simulink library "LibDBC_SCU_ch1"  (R2024b)
settings: Solver=VariableStepAuto  StartTime=0.0  StopTime=10.0  RelTol=1e-3
undefined symbols (not defined in the file): bit_packing, bit_unpacking, IO_Blk_Lib_TTC500, IO_CAN_ConfigMsg, IO_CAN_ReadMsg
libraries: simulink x59, IOBlock_Library_TTC580 x32
(part 20 of 21)

== system LibDBC_SCU_ch1/mBMS_Cell_Info_Slave2/IO_CAN_ReadMsg ==
  handle : Inport
  Enable : EnablePort
  IO_CAN_ReadMsg : IOBlock_Library_TTC580/CAN  Blocks TTC580 IOlib/ReadMsg_CAN/IO_CAN_ReadMsg  SampleTime=-1  ttlib=IO_Blk_Lib_TTC500  ttDescription=IO_CAN_ReadMsg  tt_iolib_version=0.19
      settings: SourceProductName=I/O Blocklibrary for TTC580
  ErrorCode : Outport  VectorParamsAs1DForOutWhenUnconnected=off
  buffer_data : Outport  Port=2  VectorParamsAs1DForOutWhenUnconnected=off
  buffer_length : Outport  Port=3  VectorParamsAs1DForOutWhenUnconnected=off
  buffer_id_format : Outport  Port=4  VectorParamsAs1DForOutWhenUnconnected=off
  buffer_id : Outport  Port=5  VectorParamsAs1DForOutWhenUnconnected=off
  wires:
  IO_CAN_ReadMsg/5 -> buffer_id/1
  IO_CAN_ReadMsg/4 -> buffer_id_format/1
  IO_CAN_ReadMsg/3 -> buffer_length/1
  IO_CAN_ReadMsg/2 -> buffer_data/1
  IO_CAN_ReadMsg/1 -> ErrorCode/1
  handle/1 -> IO_CAN_ReadMsg/1

== system LibDBC_SCU_ch1/mBMS_Cell_Info_Slave2/Trigger_Block ==
  Compare To Constant : simulink/Logic and Bit Operations/Compare To Constant  relop===  const=trigger_offset  OutDataTypeStr=boolean  ZeroCross=off
  Counter Limited : simulink/Sources/Counter Limited  uplimit=max(derate - 1,0)  tsamp=-1
  Trigger : Outport  VectorParamsAs1DForOutWhenUnconnected=off
  wires:
  Compare To Constant/1 -> Trigger/1
  Counter Limited/1 -> Compare To Constant/1

== system LibDBC_SCU_ch1/mBMS_Cell_Info_Slave2/bit_unpacking1 ==
  Data_in : Inport
  bit_unpacking_s : S-Function  FunctionName=bit_unpacking_s  Parameters=SampleTime,Endianness,Format,Inversion,Startbit,Width_bits,Factor,Offset  SFunctionDeploymentMode=off  EnableBusSupport=off
  Data_out : Outport  VectorParamsAs1DForOutWhenUnconnected=off
  wires:
  Data_in/1 -> bit_unpacking_s/1
  bit_unpacking_s/1 -> Data_out/1

== system LibDBC_SCU_ch1/mBMS_Cell_Info_Slave2/bit_unpacking2 ==
  Data_in : Inport
  bit_unpacking_s : S-Function  FunctionName=bit_unpacking_s  Parameters=SampleTime,Endianness,Format,Inversion,Startbit,Width_bits,Factor,Offset  SFunctionDeploymentMode=off  EnableBusSupport=off
  Data_out : Outport  VectorParamsAs1DForOutWhenUnconnected=off
  wires:
  Data_in/1 -> bit_unpacking_s/1
  bit_unpacking_s/1 -> Data_out/1

== system LibDBC_SCU_ch1/mBMS_Cell_Info_Slave2/bit_unpacking3 ==
  Data_in : Inport
  bit_unpacking_s : S-Function  FunctionName=bit_unpacking_s  Parameters=SampleTime,Endianness,Format,Inversion,Startbit,Width_bits,Factor,Offset  SFunctionDeploymentMode=off  EnableBusSupport=off
  Data_out : Outport  VectorParamsAs1DForOutWhenUnconnected=off
  wires:
  Data_in/1 -> bit_unpacking_s/1
  bit_unpacking_s/1 -> Data_out/1

== system LibDBC_SCU_ch1/mBMS_Cell_Info_Slave2/bit_unpacking4 ==
  Data_in : Inport
  bit_unpacking_s : S-Function  FunctionName=bit_unpacking_s  Parameters=SampleTime,Endianness,Format,Inversion,Startbit,Width_bits,Factor,Offset  SFunctionDeploymentMode=off  EnableBusSupport=off
  Data_out : Outport  VectorParamsAs1DForOutWhenUnconnected=off
  wires:
  Data_in/1 -> bit_unpacking_s/1
  bit_unpacking_s/1 -> Data_out/1

== system LibDBC_SCU_ch1/mBMS_Cell_Info_Slave2/bit_unpacking5 ==
  Data_in : Inport
  bit_unpacking_s : S-Function  FunctionName=bit_unpacking_s  Parameters=SampleTime,Endianness,Format,Inversion,Startbit,Width_bits,Factor,Offset  SFunctionDeploymentMode=off  EnableBusSupport=off
  Data_out : Outport  VectorParamsAs1DForOutWhenUnconnected=off
  wires:
  Data_in/1 -> bit_unpacking_s/1
  bit_unpacking_s/1 -> Data_out/1

== system LibDBC_SCU_ch1/mBMS_Cell_Info_Slave3/IO_CAN_ConfigMsg ==
  IO_CAN_ConfigMsg_s : S-Function  FunctionName=IO_CAN_ConfigMsg_s  Parameters=SampleTime,channel,mode,id_format,id,ac_mask  SFunctionDeploymentMode=off  EnableBusSupport=off
  ErrorCode : Outport  VectorParamsAs1DForOutWhenUnconnected=off
  handle : Outport  Port=2  VectorParamsAs1DForOutWhenUnconnected=off
  wires:
  IO_CAN_ConfigMsg_s/2 -> handle/1
  IO_CAN_ConfigMsg_s/1 -> ErrorCode/1

== system LibDBC_SCU_ch1/mBMS_Cell_Info_Slave3/IO_CAN_ReadMsg ==
  handle : Inport
  Enable : EnablePort
  IO_CAN_ReadMsg : IOBlock_Library_TTC580/CAN  Blocks TTC580 IOlib/ReadMsg_CAN/IO_CAN_ReadMsg  SampleTime=-1  ttlib=IO_Blk_Lib_TTC500  ttDescription=IO_CAN_ReadMsg  tt_iolib_version=0.19
      settings: SourceProductName=I/O Blocklibrary for TTC580
  ErrorCode : Outport  VectorParamsAs1DForOutWhenUnconnected=off
  buffer_data : Outport  Port=2  VectorParamsAs1DForOutWhenUnconnected=off
  buffer_length : Outport  Port=3  VectorParamsAs1DForOutWhenUnconnected=off
  buffer_id_format : Outport  Port=4  VectorParamsAs1DForOutWhenUnconnected=off
  buffer_id : Outport  Port=5  VectorParamsAs1DForOutWhenUnconnected=off
  wires:
  IO_CAN_ReadMsg/5 -> buffer_id/1
  IO_CAN_ReadMsg/4 -> buffer_id_format/1
  IO_CAN_ReadMsg/3 -> buffer_length/1
  IO_CAN_ReadMsg/2 -> buffer_data/1
  IO_CAN_ReadMsg/1 -> ErrorCode/1
  handle/1 -> IO_CAN_ReadMsg/1

== system LibDBC_SCU_ch1/mBMS_Cell_Info_Slave3/Trigger_Block ==
  Compare To Constant : simulink/Logic and Bit Operations/Compare To Constant  relop===  const=trigger_offset  OutDataTypeStr=boolean  ZeroCross=off
  Counter Limited : simulink/Sources/Counter Limited  uplimit=max(derate - 1,0)  tsamp=-1
  Trigger : Outport  VectorParamsAs1DForOutWhenUnconnected=off
  wires:
  Compare To Constant/1 -> Trigger/1
  Counter Limited/1 -> Compare To Constant/1

== system LibDBC_SCU_ch1/mBMS_Cell_Info_Slave3/bit_unpacking1 ==
  Data_in : Inport
  bit_unpacking_s : S-Function  FunctionName=bit_unpacking_s  Parameters=SampleTime,Endianness,Format,Inversion,Startbit,Width_bits,Factor,Offset  SFunctionDeploymentMode=off  EnableBusSupport=off
  Data_out : Outport  VectorParamsAs1DForOutWhenUnconnected=off
  wires:
  Data_in/1 -> bit_unpacking_s/1
  bit_unpacking_s/1 -> Data_out/1

== system LibDBC_SCU_ch1/mBMS_Cell_Info_Slave3/bit_unpacking2 ==
  Data_in : Inport
  bit_unpacking_s : S-Function  FunctionName=bit_unpacking_s  Parameters=SampleTime,Endianness,Format,Inversion,Startbit,Width_bits,Factor,Offset  SFunctionDeploymentMode=off  EnableBusSupport=off
  Data_out : Outport  VectorParamsAs1DForOutWhenUnconnected=off
  wires:
  Data_in/1 -> bit_unpacking_s/1
  bit_unpacking_s/1 -> Data_out/1

== system LibDBC_SCU_ch1/mBMS_Cell_Info_Slave3/bit_unpacking3 ==
  Data_in : Inport
  bit_unpacking_s : S-Function  FunctionName=bit_unpacking_s  Parameters=SampleTime,Endianness,Format,Inversion,Startbit,Width_bits,Factor,Offset  SFunctionDeploymentMode=off  EnableBusSupport=off
  Data_out : Outport  VectorParamsAs1DForOutWhenUnconnected=off
  wires:
  Data_in/1 -> bit_unpacking_s/1
  bit_unpacking_s/1 -> Data_out/1

== system LibDBC_SCU_ch1/mBMS_Cell_Info_Slave3/bit_unpacking4 ==
  Data_in : Inport
  bit_unpacking_s : S-Function  FunctionName=bit_unpacking_s  Parameters=SampleTime,Endianness,Format,Inversion,Startbit,Width_bits,Factor,Offset  SFunctionDeploymentMode=off  EnableBusSupport=off
  Data_out : Outport  VectorParamsAs1DForOutWhenUnconnected=off
  wires:
  Data_in/1 -> bit_unpacking_s/1
  bit_unpacking_s/1 -> Data_out/1

== system LibDBC_SCU_ch1/mBMS_Cell_Info_Slave3/bit_unpacking5 ==
  Data_in : Inport
  bit_unpacking_s : S-Function  FunctionName=bit_unpacking_s  Parameters=SampleTime,Endianness,Format,Inversion,Startbit,Width_bits,Factor,Offset  SFunctionDeploymentMode=off  EnableBusSupport=off
  Data_out : Outport  VectorParamsAs1DForOutWhenUnconnected=off
  wires:
  Data_in/1 -> bit_unpacking_s/1
  bit_unpacking_s/1 -> Data_out/1

== system LibDBC_SCU_ch1/mBMS_Cell_Info_Slave4/IO_CAN_ConfigMsg ==
  IO_CAN_ConfigMsg_s : S-Function  FunctionName=IO_CAN_ConfigMsg_s  Parameters=SampleTime,channel,mode,id_format,id,ac_mask  SFunctionDeploymentMode=off  EnableBusSupport=off
  ErrorCode : Outport  VectorParamsAs1DForOutWhenUnconnected=off
  handle : Outport  Port=2  VectorParamsAs1DForOutWhenUnconnected=off
  wires:
  IO_CAN_ConfigMsg_s/2 -> handle/1
  IO_CAN_ConfigMsg_s/1 -> ErrorCode/1

== system LibDBC_SCU_ch1/mBMS_Cell_Info_Slave4/IO_CAN_ReadMsg ==
  handle : Inport
  Enable : EnablePort
  IO_CAN_ReadMsg : IOBlock_Library_TTC580/CAN  Blocks TTC580 IOlib/ReadMsg_CAN/IO_CAN_ReadMsg  SampleTime=-1  ttlib=IO_Blk_Lib_TTC500  ttDescription=IO_CAN_ReadMsg  tt_iolib_version=0.19
      settings: SourceProductName=I/O Blocklibrary for TTC580
  ErrorCode : Outport  VectorParamsAs1DForOutWhenUnconnected=off
  buffer_data : Outport  Port=2  VectorParamsAs1DForOutWhenUnconnected=off
  buffer_length : Outport  Port=3  VectorParamsAs1DForOutWhenUnconnected=off
  buffer_id_format : Outport  Port=4  VectorParamsAs1DForOutWhenUnconnected=off
  buffer_id : Outport  Port=5  VectorParamsAs1DForOutWhenUnconnected=off
  wires:
  IO_CAN_ReadMsg/5 -> buffer_id/1
  IO_CAN_ReadMsg/4 -> buffer_id_format/1
  IO_CAN_ReadMsg/3 -> buffer_length/1
  IO_CAN_ReadMsg/2 -> buffer_data/1
  IO_CAN_ReadMsg/1 -> ErrorCode/1
  handle/1 -> IO_CAN_ReadMsg/1

== system LibDBC_SCU_ch1/mBMS_Cell_Info_Slave4/Trigger_Block ==
  Compare To Constant : simulink/Logic and Bit Operations/Compare To Constant  relop===  const=trigger_offset  OutDataTypeStr=boolean  ZeroCross=off
  Counter Limited : simulink/Sources/Counter Limited  uplimit=max(derate - 1,0)  tsamp=-1
  Trigger : Outport  VectorParamsAs1DForOutWhenUnconnected=off
  wires:
  Compare To Constant/1 -> Trigger/1
  Counter Limited/1 -> Compare To Constant/1

== system LibDBC_SCU_ch1/mBMS_Cell_Info_Slave4/bit_unpacking1 ==
  Data_in : Inport
  bit_unpacking_s : S-Function  FunctionName=bit_unpacking_s  Parameters=SampleTime,Endianness,Format,Inversion,Startbit,Width_bits,Factor,Offset  SFunctionDeploymentMode=off  EnableBusSupport=off
  Data_out : Outport  VectorParamsAs1DForOutWhenUnconnected=off
  wires:
  Data_in/1 -> bit_unpacking_s/1
  bit_unpacking_s/1 -> Data_out/1

== system LibDBC_SCU_ch1/mBMS_Cell_Info_Slave4/bit_unpacking2 ==
  Data_in : Inport
  bit_unpacking_s : S-Function  FunctionName=bit_unpacking_s  Parameters=SampleTime,Endianness,Format,Inversion,Startbit,Width_bits,Factor,Offset  SFunctionDeploymentMode=off  EnableBusSupport=off
  Data_out : Outport  VectorParamsAs1DForOutWhenUnconnected=off
  wires:
  Data_in/1 -> bit_unpacking_s/1
  bit_unpacking_s/1 -> Data_out/1

== system LibDBC_SCU_ch1/mBMS_Cell_Info_Slave4/bit_unpacking3 ==
  Data_in : Inport
  bit_unpacking_s : S-Function  FunctionName=bit_unpacking_s  Parameters=SampleTime,Endianness,Format,Inversion,Startbit,Width_bits,Factor,Offset  SFunctionDeploymentMode=off  EnableBusSupport=off
  Data_out : Outport  VectorParamsAs1DForOutWhenUnconnected=off
  wires:
  Data_in/1 -> bit_unpacking_s/1
  bit_unpacking_s/1 -> Data_out/1

== system LibDBC_SCU_ch1/mBMS_Cell_Info_Slave4/bit_unpacking4 ==
  Data_in : Inport
  bit_unpacking_s : S-Function  FunctionName=bit_unpacking_s  Parameters=SampleTime,Endianness,Format,Inversion,Startbit,Width_bits,Factor,Offset  SFunctionDeploymentMode=off  EnableBusSupport=off
  Data_out : Outport  VectorParamsAs1DForOutWhenUnconnected=off
  wires:
  Data_in/1 -> bit_unpacking_s/1
  bit_unpacking_s/1 -> Data_out/1

== system LibDBC_SCU_ch1/mBMS_Cell_Info_Slave4/bit_unpacking5 ==
  Data_in : Inport
  bit_unpacking_s : S-Function  FunctionName=bit_unpacking_s  Parameters=SampleTime,Endianness,Format,Inversion,Startbit,Width_bits,Factor,Offset  SFunctionDeploymentMode=off  EnableBusSupport=off
  Data_out : Outport  VectorParamsAs1DForOutWhenUnconnected=off
  wires:
  Data_in/1 -> bit_unpacking_s/1
  bit_unpacking_s/1 -> Data_out/1

== system LibDBC_SCU_ch1/mBMS_Cell_Info_Slave5/IO_CAN_ConfigMsg ==
  IO_CAN_ConfigMsg_s : S-Function  FunctionName=IO_CAN_ConfigMsg_s  Parameters=SampleTime,channel,mode,id_format,id,ac_mask  SFunctionDeploymentMode=off  EnableBusSupport=off
  ErrorCode : Outport  VectorParamsAs1DForOutWhenUnconnected=off
  handle : Outport  Port=2  VectorParamsAs1DForOutWhenUnconnected=off
  wires:
  IO_CAN_ConfigMsg_s/2 -> handle/1
  IO_CAN_ConfigMsg_s/1 -> ErrorCode/1

== system LibDBC_SCU_ch1/mBMS_Cell_Info_Slave5/IO_CAN_ReadMsg ==
  handle : Inport
  Enable : EnablePort
  IO_CAN_ReadMsg : IOBlock_Library_TTC580/CAN  Blocks TTC580 IOlib/ReadMsg_CAN/IO_CAN_ReadMsg  SampleTime=-1  ttlib=IO_Blk_Lib_TTC500  ttDescription=IO_CAN_ReadMsg  tt_iolib_version=0.19
      settings: SourceProductName=I/O Blocklibrary for TTC580
  ErrorCode : Outport  VectorParamsAs1DForOutWhenUnconnected=off
  buffer_data : Outport  Port=2  VectorParamsAs1DForOutWhenUnconnected=off
  buffer_length : Outport  Port=3  VectorParamsAs1DForOutWhenUnconnected=off
  buffer_id_format : Outport  Port=4  VectorParamsAs1DForOutWhenUnconnected=off
  buffer_id : Outport  Port=5  VectorParamsAs1DForOutWhenUnconnected=off
  wires:
  IO_CAN_ReadMsg/5 -> buffer_id/1
  IO_CAN_ReadMsg/4 -> buffer_id_format/1
  IO_CAN_ReadMsg/3 -> buffer_length/1
  IO_CAN_ReadMsg/2 -> buffer_data/1
  IO_CAN_ReadMsg/1 -> ErrorCode/1
  handle/1 -> IO_CAN_ReadMsg/1

== system LibDBC_SCU_ch1/mBMS_Cell_Info_Slave5/Trigger_Block ==
  Compare To Constant : simulink/Logic and Bit Operations/Compare To Constant  relop===  const=trigger_offset  OutDataTypeStr=boolean  ZeroCross=off
  Counter Limited : simulink/Sources/Counter Limited  uplimit=max(derate - 1,0)  tsamp=-1
  Trigger : Outport  VectorParamsAs1DForOutWhenUnconnected=off
  wires:
  Compare To Constant/1 -> Trigger/1
  Counter Limited/1 -> Compare To Constant/1

== system LibDBC_SCU_ch1/mBMS_Cell_Info_Slave5/bit_unpacking1 ==
  Data_in : Inport
  bit_unpacking_s : S-Function  FunctionName=bit_unpacking_s  Parameters=SampleTime,Endianness,Format,Inversion,Startbit,Width_bits,Factor,Offset  SFunctionDeploymentMode=off  EnableBusSupport=off
  Data_out : Outport  VectorParamsAs1DForOutWhenUnconnected=off
  wires:
  Data_in/1 -> bit_unpacking_s/1
  bit_unpacking_s/1 -> Data_out/1

== system LibDBC_SCU_ch1/mBMS_Cell_Info_Slave5/bit_unpacking2 ==
  Data_in : Inport
  bit_unpacking_s : S-Function  FunctionName=bit_unpacking_s  Parameters=SampleTime,Endianness,Format,Inversion,Startbit,Width_bits,Factor,Offset  SFunctionDeploymentMode=off  EnableBusSupport=off
  Data_out : Outport  VectorParamsAs1DForOutWhenUnconnected=off
  wires:
  Data_in/1 -> bit_unpacking_s/1
  bit_unpacking_s/1 -> Data_out/1

== system LibDBC_SCU_ch1/mBMS_Cell_Info_Slave5/bit_unpacking3 ==
  Data_in : Inport
  bit_unpacking_s : S-Function  FunctionName=bit_unpacking_s  Parameters=SampleTime,Endianness,Format,Inversion,Startbit,Width_bits,Factor,Offset  SFunctionDeploymentMode=off  EnableBusSupport=off
  Data_out : Outport  VectorParamsAs1DForOutWhenUnconnected=off
  wires:
  Data_in/1 -> bit_unpacking_s/1
  bit_unpacking_s/1 -> Data_out/1

== system LibDBC_SCU_ch1/mBMS_Cell_Info_Slave5/bit_unpacking4 ==
  Data_in : Inport
  bit_unpacking_s : S-Function  FunctionName=bit_unpacking_s  Parameters=SampleTime,Endianness,Format,Inversion,Startbit,Width_bits,Factor,Offset  SFunctionDeploymentMode=off  EnableBusSupport=off
  Data_out : Outport  VectorParamsAs1DForOutWhenUnconnected=off
  wires:
  Data_in/1 -> bit_unpacking_s/1
  bit_unpacking_s/1 -> Data_out/1

== system LibDBC_SCU_ch1/mBMS_Cell_Info_Slave5/bit_unpacking5 ==
  Data_in : Inport
  bit_unpacking_s : S-Function  FunctionName=bit_unpacking_s  Parameters=SampleTime,Endianness,Format,Inversion,Startbit,Width_bits,Factor,Offset  SFunctionDeploymentMode=off  EnableBusSupport=off
  Data_out : Outport  VectorParamsAs1DForOutWhenUnconnected=off
  wires:
  Data_in/1 -> bit_unpacking_s/1
  bit_unpacking_s/1 -> Data_out/1

== system LibDBC_SCU_ch1/mBMS_Cell_Info_Slave6/IO_CAN_ConfigMsg ==
  IO_CAN_ConfigMsg_s : S-Function  FunctionName=IO_CAN_ConfigMsg_s  Parameters=SampleTime,channel,mode,id_format,id,ac_mask  SFunctionDeploymentMode=off  EnableBusSupport=off
  ErrorCode : Outport  VectorParamsAs1DForOutWhenUnconnected=off
  handle : Outport  Port=2  VectorParamsAs1DForOutWhenUnconnected=off
  wires:
  IO_CAN_ConfigMsg_s/2 -> handle/1
  IO_CAN_ConfigMsg_s/1 -> ErrorCode/1

== system LibDBC_SCU_ch1/mBMS_Cell_Info_Slave6/IO_CAN_ReadMsg ==
  handle : Inport
  Enable : EnablePort
  IO_CAN_ReadMsg : IOBlock_Library_TTC580/CAN  Blocks TTC580 IOlib/ReadMsg_CAN/IO_CAN_ReadMsg  SampleTime=-1  ttlib=IO_Blk_Lib_TTC500  ttDescription=IO_CAN_ReadMsg  tt_iolib_version=0.19
      settings: SourceProductName=I/O Blocklibrary for TTC580
  ErrorCode : Outport  VectorParamsAs1DForOutWhenUnconnected=off
  buffer_data : Outport  Port=2  VectorParamsAs1DForOutWhenUnconnected=off
  buffer_length : Outport  Port=3  VectorParamsAs1DForOutWhenUnconnected=off
  buffer_id_format : Outport  Port=4  VectorParamsAs1DForOutWhenUnconnected=off
  buffer_id : Outport  Port=5  VectorParamsAs1DForOutWhenUnconnected=off
  wires:
  IO_CAN_ReadMsg/5 -> buffer_id/1
  IO_CAN_ReadMsg/4 -> buffer_id_format/1
  IO_CAN_ReadMsg/3 -> buffer_length/1
  IO_CAN_ReadMsg/2 -> buffer_data/1
  IO_CAN_ReadMsg/1 -> ErrorCode/1
  handle/1 -> IO_CAN_ReadMsg/1

== system LibDBC_SCU_ch1/mBMS_Cell_Info_Slave6/Trigger_Block ==
  Compare To Constant : simulink/Logic and Bit Operations/Compare To Constant  relop===  const=trigger_offset  OutDataTypeStr=boolean  ZeroCross=off
  Counter Limited : simulink/Sources/Counter Limited  uplimit=max(derate - 1,0)  tsamp=-1
  Trigger : Outport  VectorParamsAs1DForOutWhenUnconnected=off
  wires:
  Compare To Constant/1 -> Trigger/1
  Counter Limited/1 -> Compare To Constant/1

== system LibDBC_SCU_ch1/mBMS_Cell_Info_Slave6/bit_unpacking1 ==
  Data_in : Inport
  bit_unpacking_s : S-Function  FunctionName=bit_unpacking_s  Parameters=SampleTime,Endianness,Format,Inversion,Startbit,Width_bits,Factor,Offset  SFunctionDeploymentMode=off  EnableBusSupport=off
  Data_out : Outport  VectorParamsAs1DForOutWhenUnconnected=off
  wires:
  Data_in/1 -> bit_unpacking_s/1
  bit_unpacking_s/1 -> Data_out/1

== system LibDBC_SCU_ch1/mBMS_Cell_Info_Slave6/bit_unpacking2 ==
  Data_in : Inport
  bit_unpacking_s : S-Function  FunctionName=bit_unpacking_s  Parameters=SampleTime,Endianness,Format,Inversion,Startbit,Width_bits,Factor,Offset  SFunctionDeploymentMode=off  EnableBusSupport=off
  Data_out : Outport  VectorParamsAs1DForOutWhenUnconnected=off
  wires:
  Data_in/1 -> bit_unpacking_s/1
  bit_unpacking_s/1 -> Data_out/1

== system LibDBC_SCU_ch1/mBMS_Cell_Info_Slave6/bit_unpacking3 ==
  Data_in : Inport
  bit_unpacking_s : S-Function  FunctionName=bit_unpacking_s  Parameters=SampleTime,Endianness,Format,Inversion,Startbit,Width_bits,Factor,Offset  SFunctionDeploymentMode=off  EnableBusSupport=off
  Data_out : Outport  VectorParamsAs1DForOutWhenUnconnected=off
  wires:
  Data_in/1 -> bit_unpacking_s/1
  bit_unpacking_s/1 -> Data_out/1

== system LibDBC_SCU_ch1/mBMS_Cell_Info_Slave6/bit_unpacking4 ==
  Data_in : Inport
  bit_unpacking_s : S-Function  FunctionName=bit_unpacking_s  Parameters=SampleTime,Endianness,Format,Inversion,Startbit,Width_bits,Factor,Offset  SFunctionDeploymentMode=off  EnableBusSupport=off
  Data_out : Outport  VectorParamsAs1DForOutWhenUnconnected=off
  wires:
  Data_in/1 -> bit_unpacking_s/1
  bit_unpacking_s/1 -> Data_out/1

== system LibDBC_SCU_ch1/mBMS_Cell_Info_Slave6/bit_unpacking5 ==
  Data_in : Inport
  bit_unpacking_s : S-Function  FunctionName=bit_unpacking_s  Parameters=SampleTime,Endianness,Format,Inversion,Startbit,Width_bits,Factor,Offset  SFunctionDeploymentMode=off  EnableBusSupport=off
  Data_out : Outport  VectorParamsAs1DForOutWhenUnconnected=off
  wires:
  Data_in/1 -> bit_unpacking_s/1
  bit_unpacking_s/1 -> Data_out/1

== system LibDBC_SCU_ch1/mBMS_Cell_Info_Slave7/IO_CAN_ConfigMsg ==
  IO_CAN_ConfigMsg_s : S-Function  FunctionName=IO_CAN_ConfigMsg_s  Parameters=SampleTime,channel,mode,id_format,id,ac_mask  SFunctionDeploymentMode=off  EnableBusSupport=off
  ErrorCode : Outport  VectorParamsAs1DForOutWhenUnconnected=off
  handle : Outport  Port=2  VectorParamsAs1DForOutWhenUnconnected=off
  wires:
  IO_CAN_ConfigMsg_s/2 -> handle/1
  IO_CAN_ConfigMsg_s/1 -> ErrorCode/1

== system LibDBC_SCU_ch1/mBMS_Cell_Info_Slave7/IO_CAN_ReadMsg ==
  handle : Inport
  Enable : EnablePort
  IO_CAN_ReadMsg : IOBlock_Library_TTC580/CAN  Blocks TTC580 IOlib/ReadMsg_CAN/IO_CAN_ReadMsg  SampleTime=-1  ttlib=IO_Blk_Lib_TTC500  ttDescription=IO_CAN_ReadMsg  tt_iolib_version=0.19
      settings: SourceProductName=I/O Blocklibrary for TTC580
  ErrorCode : Outport  VectorParamsAs1DForOutWhenUnconnected=off
  buffer_data : Outport  Port=2  VectorParamsAs1DForOutWhenUnconnected=off
  buffer_length : Outport  Port=3  VectorParamsAs1DForOutWhenUnconnected=off
  buffer_id_format : Outport  Port=4  VectorParamsAs1DForOutWhenUnconnected=off
  buffer_id : Outport  Port=5  VectorParamsAs1DForOutWhenUnconnected=off
  wires:
  IO_CAN_ReadMsg/5 -> buffer_id/1
  IO_CAN_ReadMsg/4 -> buffer_id_format/1
  IO_CAN_ReadMsg/3 -> buffer_length/1
  IO_CAN_ReadMsg/2 -> buffer_data/1
  IO_CAN_ReadMsg/1 -> ErrorCode/1
  handle/1 -> IO_CAN_ReadMsg/1

== system LibDBC_SCU_ch1/mBMS_Cell_Info_Slave7/Trigger_Block ==
  Compare To Constant : simulink/Logic and Bit Operations/Compare To Constant  relop===  const=trigger_offset  OutDataTypeStr=boolean  ZeroCross=off
  Counter Limited : simulink/Sources/Counter Limited  uplimit=max(derate - 1,0)  tsamp=-1
  Trigger : Outport  VectorParamsAs1DForOutWhenUnconnected=off
  wires:
  Compare To Constant/1 -> Trigger/1
  Counter Limited/1 -> Compare To Constant/1

== system LibDBC_SCU_ch1/mBMS_Cell_Info_Slave7/bit_unpacking1 ==
  Data_in : Inport
  bit_unpacking_s : S-Function  FunctionName=bit_unpacking_s  Parameters=SampleTime,Endianness,Format,Inversion,Startbit,Width_bits,Factor,Offset  SFunctionDeploymentMode=off  EnableBusSupport=off
  Data_out : Outport  VectorParamsAs1DForOutWhenUnconnected=off
  wires:
  Data_in/1 -> bit_unpacking_s/1
  bit_unpacking_s/1 -> Data_out/1

== system LibDBC_SCU_ch1/mBMS_Cell_Info_Slave7/bit_unpacking2 ==
  Data_in : Inport
  bit_unpacking_s : S-Function  FunctionName=bit_unpacking_s  Parameters=SampleTime,Endianness,Format,Inversion,Startbit,Width_bits,Factor,Offset  SFunctionDeploymentMode=off  EnableBusSupport=off
  Data_out : Outport  VectorParamsAs1DForOutWhenUnconnected=off
  wires:
  Data_in/1 -> bit_unpacking_s/1
  bit_unpacking_s/1 -> Data_out/1

== system LibDBC_SCU_ch1/mBMS_Cell_Info_Slave7/bit_unpacking3 ==
  Data_in : Inport
  bit_unpacking_s : S-Function  FunctionName=bit_unpacking_s  Parameters=SampleTime,Endianness,Format,Inversion,Startbit,Width_bits,Factor,Offset  SFunctionDeploymentMode=off  EnableBusSupport=off
  Data_out : Outport  VectorParamsAs1DForOutWhenUnconnected=off
  wires:
  Data_in/1 -> bit_unpacking_s/1
  bit_unpacking_s/1 -> Data_out/1

== system LibDBC_SCU_ch1/mBMS_Cell_Info_Slave7/bit_unpacking4 ==
  Data_in : Inport
  bit_unpacking_s : S-Function  FunctionName=bit_unpacking_s  Parameters=SampleTime,Endianness,Format,Inversion,Startbit,Width_bits,Factor,Offset  SFunctionDeploymentMode=off  EnableBusSupport=off
  Data_out : Outport  VectorParamsAs1DForOutWhenUnconnected=off
  wires:
  Data_in/1 -> bit_unpacking_s/1
  bit_unpacking_s/1 -> Data_out/1

== system LibDBC_SCU_ch1/mBMS_Cell_Info_Slave7/bit_unpacking5 ==
  Data_in : Inport
  bit_unpacking_s : S-Function  FunctionName=bit_unpacking_s  Parameters=SampleTime,Endianness,Format,Inversion,Startbit,Width_bits,Factor,Offset  SFunctionDeploymentMode=off  EnableBusSupport=off
  Data_out : Outport  VectorParamsAs1DForOutWhenUnconnected=off
  wires:
  Data_in/1 -> bit_unpacking_s/1
  bit_unpacking_s/1 -> Data_out/1

== system LibDBC_SCU_ch1/mBMS_FuncSTAT/IO_CAN_ConfigMsg ==
  IO_CAN_ConfigMsg_s : S-Function  FunctionName=IO_CAN_ConfigMsg_s  Parameters=SampleTime,channel,mode,id_format,id,ac_mask  SFunctionDeploymentMode=off  EnableBusSupport=off
  ErrorCode : Outport  VectorParamsAs1DForOutWhenUnconnected=off
  handle : Outport  Port=2  VectorParamsAs1DForOutWhenUnconnected=off
  wires:
  IO_CAN_ConfigMsg_s/2 -> handle/1
  IO_CAN_ConfigMsg_s/1 -> ErrorCode/1

== system LibDBC_SCU_ch1/mBMS_FuncSTAT/IO_CAN_ReadMsg ==
  handle : Inport
  Enable : EnablePort
  IO_CAN_ReadMsg : IOBlock_Library_TTC580/CAN  Blocks TTC580 IOlib/ReadMsg_CAN/IO_CAN_ReadMsg  SampleTime=-1  ttlib=IO_Blk_Lib_TTC500  ttDescription=IO_CAN_ReadMsg  tt_iolib_version=0.19
      settings: SourceProductName=I/O Blocklibrary for TTC580
  ErrorCode : Outport  VectorParamsAs1DForOutWhenUnconnected=off
  buffer_data : Outport  Port=2  VectorParamsAs1DForOutWhenUnconnected=off
  buffer_length : Outport  Port=3  VectorParamsAs1DForOutWhenUnconnected=off
  buffer_id_format : Outport  Port=4  VectorParamsAs1DForOutWhenUnconnected=off
  buffer_id : Outport  Port=5  VectorParamsAs1DForOutWhenUnconnected=off
  wires:
  IO_CAN_ReadMsg/5 -> buffer_id/1
  IO_CAN_ReadMsg/4 -> buffer_id_format/1
  IO_CAN_ReadMsg/3 -> buffer_length/1
  IO_CAN_ReadMsg/2 -> buffer_data/1
  IO_CAN_ReadMsg/1 -> ErrorCode/1
  handle/1 -> IO_CAN_ReadMsg/1

== system LibDBC_SCU_ch1/mBMS_FuncSTAT/Trigger_Block ==
  Compare To Constant : simulink/Logic and Bit Operations/Compare To Constant  relop===  const=trigger_offset  OutDataTypeStr=boolean  ZeroCross=off
  Counter Limited : simulink/Sources/Counter Limited  uplimit=max(derate - 1,0)  tsamp=-1
  Trigger : Outport  VectorParamsAs1DForOutWhenUnconnected=off
  wires:
  Compare To Constant/1 -> Trigger/1
  Counter Limited/1 -> Compare To Constant/1

== system LibDBC_SCU_ch1/mBMS_FuncSTAT/bit_unpacking1 ==
  Data_in : Inport
  bit_unpacking_s : S-Function  FunctionName=bit_unpacking_s  Parameters=SampleTime,Endianness,Format,Inversion,Startbit,Width_bits,Factor,Offset  SFunctionDeploymentMode=off  EnableBusSupport=off
  Data_out : Outport  VectorParamsAs1DForOutWhenUnconnected=off
  wires:
  Data_in/1 -> bit_unpacking_s/1
  bit_unpacking_s/1 -> Data_out/1

== system LibDBC_SCU_ch1/mBMS_FuncSTAT/bit_unpacking10 ==
  Data_in : Inport
  bit_unpacking_s : S-Function  FunctionName=bit_unpacking_s  Parameters=SampleTime,Endianness,Format,Inversion,Startbit,Width_bits,Factor,Offset  SFunctionDeploymentMode=off  EnableBusSupport=off
  Data_out : Outport  VectorParamsAs1DForOutWhenUnconnected=off
  wires:
  Data_in/1 -> bit_unpacking_s/1
  bit_unpacking_s/1 -> Data_out/1

== system LibDBC_SCU_ch1/mBMS_FuncSTAT/bit_unpacking11 ==
  Data_in : Inport
  bit_unpacking_s : S-Function  FunctionName=bit_unpacking_s  Parameters=SampleTime,Endianness,Format,Inversion,Startbit,Width_bits,Factor,Offset  SFunctionDeploymentMode=off  EnableBusSupport=off
  Data_out : Outport  VectorParamsAs1DForOutWhenUnconnected=off
  wires:
  Data_in/1 -> bit_unpacking_s/1
  bit_unpacking_s/1 -> Data_out/1

== system LibDBC_SCU_ch1/mBMS_FuncSTAT/bit_unpacking12 ==
  Data_in : Inport
  bit_unpacking_s : S-Function  FunctionName=bit_unpacking_s  Parameters=SampleTime,Endianness,Format,Inversion,Startbit,Width_bits,Factor,Offset  SFunctionDeploymentMode=off  EnableBusSupport=off
  Data_out : Outport  VectorParamsAs1DForOutWhenUnconnected=off
  wires:
  Data_in/1 -> bit_unpacking_s/1
  bit_unpacking_s/1 -> Data_out/1

== system LibDBC_SCU_ch1/mBMS_FuncSTAT/bit_unpacking13 ==
  Data_in : Inport
  bit_unpacking_s : S-Function  FunctionName=bit_unpacking_s  Parameters=SampleTime,Endianness,Format,Inversion,Startbit,Width_bits,Factor,Offset  SFunctionDeploymentMode=off  EnableBusSupport=off
  Data_out : Outport  VectorParamsAs1DForOutWhenUnconnected=off
  wires:
  Data_in/1 -> bit_unpacking_s/1
  bit_unpacking_s/1 -> Data_out/1

== system LibDBC_SCU_ch1/mBMS_FuncSTAT/bit_unpacking14 ==
  Data_in : Inport
  bit_unpacking_s : S-Function  FunctionName=bit_unpacking_s  Parameters=SampleTime,Endianness,Format,Inversion,Startbit,Width_bits,Factor,Offset  SFunctionDeploymentMode=off  EnableBusSupport=off
  Data_out : Outport  VectorParamsAs1DForOutWhenUnconnected=off
  wires:
  Data_in/1 -> bit_unpacking_s/1
  bit_unpacking_s/1 -> Data_out/1

== system LibDBC_SCU_ch1/mBMS_FuncSTAT/bit_unpacking15 ==
  Data_in : Inport
  bit_unpacking_s : S-Function  FunctionName=bit_unpacking_s  Parameters=SampleTime,Endianness,Format,Inversion,Startbit,Width_bits,Factor,Offset  SFunctionDeploymentMode=off  EnableBusSupport=off
  Data_out : Outport  VectorParamsAs1DForOutWhenUnconnected=off
  wires:
  Data_in/1 -> bit_unpacking_s/1
  bit_unpacking_s/1 -> Data_out/1

== system LibDBC_SCU_ch1/mBMS_FuncSTAT/bit_unpacking16 ==
  Data_in : Inport
  bit_unpacking_s : S-Function  FunctionName=bit_unpacking_s  Parameters=SampleTime,Endianness,Format,Inversion,Startbit,Width_bits,Factor,Offset  SFunctionDeploymentMode=off  EnableBusSupport=off
  Data_out : Outport  VectorParamsAs1DForOutWhenUnconnected=off
  wires:
  Data_in/1 -> bit_unpacking_s/1
  bit_unpacking_s/1 -> Data_out/1

== system LibDBC_SCU_ch1/mBMS_FuncSTAT/bit_unpacking17 ==
  Data_in : Inport
  bit_unpacking_s : S-Function  FunctionName=bit_unpacking_s  Parameters=SampleTime,Endianness,Format,Inversion,Startbit,Width_bits,Factor,Offset  SFunctionDeploymentMode=off  EnableBusSupport=off
  Data_out : Outport  VectorParamsAs1DForOutWhenUnconnected=off
  wires:
  Data_in/1 -> bit_unpacking_s/1
  bit_unpacking_s/1 -> Data_out/1

== system LibDBC_SCU_ch1/mBMS_FuncSTAT/bit_unpacking18 ==
  Data_in : Inport
  bit_unpacking_s : S-Function  FunctionName=bit_unpacking_s  Parameters=SampleTime,Endianness,Format,Inversion,Startbit,Width_bits,Factor,Offset  SFunctionDeploymentMode=off  EnableBusSupport=off
  Data_out : Outport  VectorParamsAs1DForOutWhenUnconnected=off
  wires:
  Data_in/1 -> bit_unpacking_s/1
  bit_unpacking_s/1 -> Data_out/1

== system LibDBC_SCU_ch1/mBMS_FuncSTAT/bit_unpacking19 ==
  Data_in : Inport
  bit_unpacking_s : S-Function  FunctionName=bit_unpacking_s  Parameters=SampleTime,Endianness,Format,Inversion,Startbit,Width_bits,Factor,Offset  SFunctionDeploymentMode=off  EnableBusSupport=off
  Data_out : Outport  VectorParamsAs1DForOutWhenUnconnected=off
  wires:
  Data_in/1 -> bit_unpacking_s/1
  bit_unpacking_s/1 -> Data_out/1

== system LibDBC_SCU_ch1/mBMS_FuncSTAT/bit_unpacking2 ==
  Data_in : Inport
  bit_unpacking_s : S-Function  FunctionName=bit_unpacking_s  Parameters=SampleTime,Endianness,Format,Inversion,Startbit,Width_bits,Factor,Offset  SFunctionDeploymentMode=off  EnableBusSupport=off
  Data_out : Outport  VectorParamsAs1DForOutWhenUnconnected=off
  wires:
  Data_in/1 -> bit_unpacking_s/1
  bit_unpacking_s/1 -> Data_out/1

== system LibDBC_SCU_ch1/mBMS_FuncSTAT/bit_unpacking20 ==
  Data_in : Inport
  bit_unpacking_s : S-Function  FunctionName=bit_unpacking_s  Parameters=SampleTime,Endianness,Format,Inversion,Startbit,Width_bits,Factor,Offset  SFunctionDeploymentMode=off  EnableBusSupport=off
  Data_out : Outport  VectorParamsAs1DForOutWhenUnconnected=off
  wires:
  Data_in/1 -> bit_unpacking_s/1
  bit_unpacking_s/1 -> Data_out/1

== system LibDBC_SCU_ch1/mBMS_FuncSTAT/bit_unpacking21 ==
  Data_in : Inport
  bit_unpacking_s : S-Function  FunctionName=bit_unpacking_s  Parameters=SampleTime,Endianness,Format,Inversion,Startbit,Width_bits,Factor,Offset  SFunctionDeploymentMode=off  EnableBusSupport=off
  Data_out : Outport  VectorParamsAs1DForOutWhenUnconnected=off
  wires:
  Data_in/1 -> bit_unpacking_s/1
  bit_unpacking_s/1 -> Data_out/1

== system LibDBC_SCU_ch1/mBMS_FuncSTAT/bit_unpacking22 ==
  Data_in : Inport
  bit_unpacking_s : S-Function  FunctionName=bit_unpacking_s  Parameters=SampleTime,Endianness,Format,Inversion,Startbit,Width_bits,Factor,Offset  SFunctionDeploymentMode=off  EnableBusSupport=off
  Data_out : Outport  VectorParamsAs1DForOutWhenUnconnected=off
  wires:
  Data_in/1 -> bit_unpacking_s/1
  bit_unpacking_s/1 -> Data_out/1

== system LibDBC_SCU_ch1/mBMS_FuncSTAT/bit_unpacking23 ==
  Data_in : Inport
  bit_unpacking_s : S-Function  FunctionName=bit_unpacking_s  Parameters=SampleTime,Endianness,Format,Inversion,Startbit,Width_bits,Factor,Offset  SFunctionDeploymentMode=off  EnableBusSupport=off
  Data_out : Outport  VectorParamsAs1DForOutWhenUnconnected=off
  wires:
  Data_in/1 -> bit_unpacking_s/1
  bit_unpacking_s/1 -> Data_out/1

== system LibDBC_SCU_ch1/mBMS_FuncSTAT/bit_unpacking24 ==
  Data_in : Inport
  bit_unpacking_s : S-Function  FunctionName=bit_unpacking_s  Parameters=SampleTime,Endianness,Format,Inversion,Startbit,Width_bits,Factor,Offset  SFunctionDeploymentMode=off  EnableBusSupport=off
  Data_out : Outport  VectorParamsAs1DForOutWhenUnconnected=off
  wires:
  Data_in/1 -> bit_unpacking_s/1
  bit_unpacking_s/1 -> Data_out/1

== system LibDBC_SCU_ch1/mBMS_FuncSTAT/bit_unpacking25 ==
  Data_in : Inport
  bit_unpacking_s : S-Function  FunctionName=bit_unpacking_s  Parameters=SampleTime,Endianness,Format,Inversion,Startbit,Width_bits,Factor,Offset  SFunctionDeploymentMode=off  EnableBusSupport=off
  Data_out : Outport  VectorParamsAs1DForOutWhenUnconnected=off
  wires:
  Data_in/1 -> bit_unpacking_s/1
  bit_unpacking_s/1 -> Data_out/1

== system LibDBC_SCU_ch1/mBMS_FuncSTAT/bit_unpacking26 ==
  Data_in : Inport
  bit_unpacking_s : S-Function  FunctionName=bit_unpacking_s  Parameters=SampleTime,Endianness,Format,Inversion,Startbit,Width_bits,Factor,Offset  SFunctionDeploymentMode=off  EnableBusSupport=off
  Data_out : Outport  VectorParamsAs1DForOutWhenUnconnected=off
  wires:
  Data_in/1 -> bit_unpacking_s/1
  bit_unpacking_s/1 -> Data_out/1

== system LibDBC_SCU_ch1/mBMS_FuncSTAT/bit_unpacking27 ==
  Data_in : Inport
  bit_unpacking_s : S-Function  FunctionName=bit_unpacking_s  Parameters=SampleTime,Endianness,Format,Inversion,Startbit,Width_bits,Factor,Offset  SFunctionDeploymentMode=off  EnableBusSupport=off
  Data_out : Outport  VectorParamsAs1DForOutWhenUnconnected=off
  wires:
  Data_in/1 -> bit_unpacking_s/1
  bit_unpacking_s/1 -> Data_out/1

== system LibDBC_SCU_ch1/mBMS_FuncSTAT/bit_unpacking28 ==
  Data_in : Inport
  bit_unpacking_s : S-Function  FunctionName=bit_unpacking_s  Parameters=SampleTime,Endianness,Format,Inversion,Startbit,Width_bits,Factor,Offset  SFunctionDeploymentMode=off  EnableBusSupport=off
  Data_out : Outport  VectorParamsAs1DForOutWhenUnconnected=off
  wires:
  Data_in/1 -> bit_unpacking_s/1
  bit_unpacking_s/1 -> Data_out/1

== system LibDBC_SCU_ch1/mBMS_FuncSTAT/bit_unpacking29 ==
  Data_in : Inport
  bit_unpacking_s : S-Function  FunctionName=bit_unpacking_s  Parameters=SampleTime,Endianness,Format,Inversion,Startbit,Width_bits,Factor,Offset  SFunctionDeploymentMode=off  EnableBusSupport=off
  Data_out : Outport  VectorParamsAs1DForOutWhenUnconnected=off
  wires:
  Data_in/1 -> bit_unpacking_s/1
  bit_unpacking_s/1 -> Data_out/1

== system LibDBC_SCU_ch1/mBMS_FuncSTAT/bit_unpacking3 ==
  Data_in : Inport
  bit_unpacking_s : S-Function  FunctionName=bit_unpacking_s  Parameters=SampleTime,Endianness,Format,Inversion,Startbit,Width_bits,Factor,Offset  SFunctionDeploymentMode=off  EnableBusSupport=off
  Data_out : Outport  VectorParamsAs1DForOutWhenUnconnected=off
  wires:
  Data_in/1 -> bit_unpacking_s/1
  bit_unpacking_s/1 -> Data_out/1

== system LibDBC_SCU_ch1/mBMS_FuncSTAT/bit_unpacking30 ==
  Data_in : Inport
  bit_unpacking_s : S-Function  FunctionName=bit_unpacking_s  Parameters=SampleTime,Endianness,Format,Inversion,Startbit,Width_bits,Factor,Offset  SFunctionDeploymentMode=off  EnableBusSupport=off
  Data_out : Outport  VectorParamsAs1DForOutWhenUnconnected=off
  wires:
  Data_in/1 -> bit_unpacking_s/1
  bit_unpacking_s/1 -> Data_out/1

== system LibDBC_SCU_ch1/mBMS_FuncSTAT/bit_unpacking31 ==
  Data_in : Inport
  bit_unpacking_s : S-Function  FunctionName=bit_unpacking_s  Parameters=SampleTime,Endianness,Format,Inversion,Startbit,Width_bits,Factor,Offset  SFunctionDeploymentMode=off  EnableBusSupport=off
  Data_out : Outport  VectorParamsAs1DForOutWhenUnconnected=off
  wires:
  Data_in/1 -> bit_unpacking_s/1
  bit_unpacking_s/1 -> Data_out/1

== system LibDBC_SCU_ch1/mBMS_FuncSTAT/bit_unpacking32 ==
  Data_in : Inport
  bit_unpacking_s : S-Function  FunctionName=bit_unpacking_s  Parameters=SampleTime,Endianness,Format,Inversion,Startbit,Width_bits,Factor,Offset  SFunctionDeploymentMode=off  EnableBusSupport=off
  Data_out : Outport  VectorParamsAs1DForOutWhenUnconnected=off
  wires:
  Data_in/1 -> bit_unpacking_s/1
  bit_unpacking_s/1 -> Data_out/1

== system LibDBC_SCU_ch1/mBMS_FuncSTAT/bit_unpacking33 ==
  Data_in : Inport
  bit_unpacking_s : S-Function  FunctionName=bit_unpacking_s  Parameters=SampleTime,Endianness,Format,Inversion,Startbit,Width_bits,Factor,Offset  SFunctionDeploymentMode=off  EnableBusSupport=off
  Data_out : Outport  VectorParamsAs1DForOutWhenUnconnected=off
  wires:
  Data_in/1 -> bit_unpacking_s/1
  bit_unpacking_s/1 -> Data_out/1

== system LibDBC_SCU_ch1/mBMS_FuncSTAT/bit_unpacking34 ==
  Data_in : Inport
  bit_unpacking_s : S-Function  FunctionName=bit_unpacking_s  Parameters=SampleTime,Endianness,Format,Inversion,Startbit,Width_bits,Factor,Offset  SFunctionDeploymentMode=off  EnableBusSupport=off
  Data_out : Outport  VectorParamsAs1DForOutWhenUnconnected=off
  wires:
  Data_in/1 -> bit_unpacking_s/1
  bit_unpacking_s/1 -> Data_out/1

== system LibDBC_SCU_ch1/mBMS_FuncSTAT/bit_unpacking35 ==
  Data_in : Inport
  bit_unpacking_s : S-Function  FunctionName=bit_unpacking_s  Parameters=SampleTime,Endianness,Format,Inversion,Startbit,Width_bits,Factor,Offset  SFunctionDeploymentMode=off  EnableBusSupport=off
  Data_out : Outport  VectorParamsAs1DForOutWhenUnconnected=off
  wires:
  Data_in/1 -> bit_unpacking_s/1
  bit_unpacking_s/1 -> Data_out/1

== system LibDBC_SCU_ch1/mBMS_FuncSTAT/bit_unpacking36 ==
  Data_in : Inport
  bit_unpacking_s : S-Function  FunctionName=bit_unpacking_s  Parameters=SampleTime,Endianness,Format,Inversion,Startbit,Width_bits,Factor,Offset  SFunctionDeploymentMode=off  EnableBusSupport=off
  Data_out : Outport  VectorParamsAs1DForOutWhenUnconnected=off
  wires:
  Data_in/1 -> bit_unpacking_s/1
  bit_unpacking_s/1 -> Data_out/1

== system LibDBC_SCU_ch1/mBMS_FuncSTAT/bit_unpacking37 ==
  Data_in : Inport
  bit_unpacking_s : S-Function  FunctionName=bit_unpacking_s  Parameters=SampleTime,Endianness,Format,Inversion,Startbit,Width_bits,Factor,Offset  SFunctionDeploymentMode=off  EnableBusSupport=off
  Data_out : Outport  VectorParamsAs1DForOutWhenUnconnected=off
  wires:
  Data_in/1 -> bit_unpacking_s/1
  bit_unpacking_s/1 -> Data_out/1

== system LibDBC_SCU_ch1/mBMS_FuncSTAT/bit_unpacking38 ==
  Data_in : Inport
  bit_unpacking_s : S-Function  FunctionName=bit_unpacking_s  Parameters=SampleTime,Endianness,Format,Inversion,Startbit,Width_bits,Factor,Offset  SFunctionDeploymentMode=off  EnableBusSupport=off
  Data_out : Outport  VectorParamsAs1DForOutWhenUnconnected=off
  wires:
  Data_in/1 -> bit_unpacking_s/1
  bit_unpacking_s/1 -> Data_out/1

== system LibDBC_SCU_ch1/mBMS_FuncSTAT/bit_unpacking39 ==
  Data_in : Inport
  bit_unpacking_s : S-Function  FunctionName=bit_unpacking_s  Parameters=SampleTime,Endianness,Format,Inversion,Startbit,Width_bits,Factor,Offset  SFunctionDeploymentMode=off  EnableBusSupport=off
  Data_out : Outport  VectorParamsAs1DForOutWhenUnconnected=off
  wires:
  Data_in/1 -> bit_unpacking_s/1
  bit_unpacking_s/1 -> Data_out/1

== system LibDBC_SCU_ch1/mBMS_FuncSTAT/bit_unpacking4 ==
  Data_in : Inport
  bit_unpacking_s : S-Function  FunctionName=bit_unpacking_s  Parameters=SampleTime,Endianness,Format,Inversion,Startbit,Width_bits,Factor,Offset  SFunctionDeploymentMode=off  EnableBusSupport=off
  Data_out : Outport  VectorParamsAs1DForOutWhenUnconnected=off
  wires:
  Data_in/1 -> bit_unpacking_s/1
  bit_unpacking_s/1 -> Data_out/1

== system LibDBC_SCU_ch1/mBMS_FuncSTAT/bit_unpacking40 ==
  Data_in : Inport
  bit_unpacking_s : S-Function  FunctionName=bit_unpacking_s  Parameters=SampleTime,Endianness,Format,Inversion,Startbit,Width_bits,Factor,Offset  SFunctionDeploymentMode=off  EnableBusSupport=off
  Data_out : Outport  VectorParamsAs1DForOutWhenUnconnected=off
  wires:
  Data_in/1 -> bit_unpacking_s/1
  bit_unpacking_s/1 -> Data_out/1

== system LibDBC_SCU_ch1/mBMS_FuncSTAT/bit_unpacking41 ==
  Data_in : Inport
  bit_unpacking_s : S-Function  FunctionName=bit_unpacking_s  Parameters=SampleTime,Endianness,Format,Inversion,Startbit,Width_bits,Factor,Offset  SFunctionDeploymentMode=off  EnableBusSupport=off
  Data_out : Outport  VectorParamsAs1DForOutWhenUnconnected=off
  wires:
  Data_in/1 -> bit_unpacking_s/1
  bit_unpacking_s/1 -> Data_out/1

== system LibDBC_SCU_ch1/mBMS_FuncSTAT/bit_unpacking42 ==
  Data_in : Inport
  bit_unpacking_s : S-Function  FunctionName=bit_unpacking_s  Parameters=SampleTime,Endianness,Format,Inversion,Startbit,Width_bits,Factor,Offset  SFunctionDeploymentMode=off  EnableBusSupport=off
  Data_out : Outport  VectorParamsAs1DForOutWhenUnconnected=off
  wires:
  Data_in/1 -> bit_unpacking_s/1
  bit_unpacking_s/1 -> Data_out/1

== system LibDBC_SCU_ch1/mBMS_FuncSTAT/bit_unpacking43 ==
  Data_in : Inport
  bit_unpacking_s : S-Function  FunctionName=bit_unpacking_s  Parameters=SampleTime,Endianness,Format,Inversion,Startbit,Width_bits,Factor,Offset  SFunctionDeploymentMode=off  EnableBusSupport=off
  Data_out : Outport  VectorParamsAs1DForOutWhenUnconnected=off
  wires:
  Data_in/1 -> bit_unpacking_s/1
  bit_unpacking_s/1 -> Data_out/1

== system LibDBC_SCU_ch1/mBMS_FuncSTAT/bit_unpacking44 ==
  Data_in : Inport
  bit_unpacking_s : S-Function  FunctionName=bit_unpacking_s  Parameters=SampleTime,Endianness,Format,Inversion,Startbit,Width_bits,Factor,Offset  SFunctionDeploymentMode=off  EnableBusSupport=off
  Data_out : Outport  VectorParamsAs1DForOutWhenUnconnected=off
  wires:
  Data_in/1 -> bit_unpacking_s/1
  bit_unpacking_s/1 -> Data_out/1

== system LibDBC_SCU_ch1/mBMS_FuncSTAT/bit_unpacking5 ==
  Data_in : Inport
  bit_unpacking_s : S-Function  FunctionName=bit_unpacking_s  Parameters=SampleTime,Endianness,Format,Inversion,Startbit,Width_bits,Factor,Offset  SFunctionDeploymentMode=off  EnableBusSupport=off
  Data_out : Outport  VectorParamsAs1DForOutWhenUnconnected=off
  wires:
  Data_in/1 -> bit_unpacking_s/1
  bit_unpacking_s/1 -> Data_out/1

== system LibDBC_SCU_ch1/mBMS_FuncSTAT/bit_unpacking6 ==
  Data_in : Inport
  bit_unpacking_s : S-Function  FunctionName=bit_unpacking_s  Parameters=SampleTime,Endianness,Format,Inversion,Startbit,Width_bits,Factor,Offset  SFunctionDeploymentMode=off  EnableBusSupport=off
  Data_out : Outport  VectorParamsAs1DForOutWhenUnconnected=off
  wires:
  Data_in/1 -> bit_unpacking_s/1
  bit_unpacking_s/1 -> Data_out/1

== system LibDBC_SCU_ch1/mBMS_FuncSTAT/bit_unpacking7 ==
  Data_in : Inport
  bit_unpacking_s : S-Function  FunctionName=bit_unpacking_s  Parameters=SampleTime,Endianness,Format,Inversion,Startbit,Width_bits,Factor,Offset  SFunctionDeploymentMode=off  EnableBusSupport=off
  Data_out : Outport  VectorParamsAs1DForOutWhenUnconnected=off
  wires:
  Data_in/1 -> bit_unpacking_s/1
  bit_unpacking_s/1 -> Data_out/1

== system LibDBC_SCU_ch1/mBMS_FuncSTAT/bit_unpacking8 ==
  Data_in : Inport
  bit_unpacking_s : S-Function  FunctionName=bit_unpacking_s  Parameters=SampleTime,Endianness,Format,Inversion,Startbit,Width_bits,Factor,Offset  SFunctionDeploymentMode=off  EnableBusSupport=off
  Data_out : Outport  VectorParamsAs1DForOutWhenUnconnected=off
  wires:
  Data_in/1 -> bit_unpacking_s/1
  bit_unpacking_s/1 -> Data_out/1

== system LibDBC_SCU_ch1/mBMS_FuncSTAT/bit_unpacking9 ==
  Data_in : Inport
  bit_unpacking_s : S-Function  FunctionName=bit_unpacking_s  Parameters=SampleTime,Endianness,Format,Inversion,Startbit,Width_bits,Factor,Offset  SFunctionDeploymentMode=off  EnableBusSupport=off
  Data_out : Outport  VectorParamsAs1DForOutWhenUnconnected=off
  wires:
  Data_in/1 -> bit_unpacking_s/1
  bit_unpacking_s/1 -> Data_out/1

== system LibDBC_SCU_ch1/mBMS_PP/IO_CAN_ConfigMsg ==
  IO_CAN_ConfigMsg_s : S-Function  FunctionName=IO_CAN_ConfigMsg_s  Parameters=SampleTime,channel,mode,id_format,id,ac_mask  SFunctionDeploymentMode=off  EnableBusSupport=off
  ErrorCode : Outport  VectorParamsAs1DForOutWhenUnconnected=off
  handle : Outport  Port=2  VectorParamsAs1DForOutWhenUnconnected=off
  wires:
  IO_CAN_ConfigMsg_s/2 -> handle/1
  IO_CAN_ConfigMsg_s/1 -> ErrorCode/1

== system LibDBC_SCU_ch1/mBMS_PP/IO_CAN_ReadMsg ==
  handle : Inport
  Enable : EnablePort
  IO_CAN_ReadMsg : IOBlock_Library_TTC580/CAN  Blocks TTC580 IOlib/ReadMsg_CAN/IO_CAN_ReadMsg  SampleTime=-1  ttlib=IO_Blk_Lib_TTC500  ttDescription=IO_CAN_ReadMsg  tt_iolib_version=0.19
      settings: SourceProductName=I/O Blocklibrary for TTC580
  ErrorCode : Outport  VectorParamsAs1DForOutWhenUnconnected=off
  buffer_data : Outport  Port=2  VectorParamsAs1DForOutWhenUnconnected=off
  buffer_length : Outport  Port=3  VectorParamsAs1DForOutWhenUnconnected=off
  buffer_id_format : Outport  Port=4  VectorParamsAs1DForOutWhenUnconnected=off
  buffer_id : Outport  Port=5  VectorParamsAs1DForOutWhenUnconnected=off
  wires:
  IO_CAN_ReadMsg/5 -> buffer_id/1
  IO_CAN_ReadMsg/4 -> buffer_id_format/1
  IO_CAN_ReadMsg/3 -> buffer_length/1
  IO_CAN_ReadMsg/2 -> buffer_data/1
  IO_CAN_ReadMsg/1 -> ErrorCode/1
  handle/1 -> IO_CAN_ReadMsg/1

== system LibDBC_SCU_ch1/mBMS_PP/Trigger_Block ==
  Compare To Constant : simulink/Logic and Bit Operations/Compare To Constant  relop===  const=trigger_offset  OutDataTypeStr=boolean  ZeroCross=off
  Counter Limited : simulink/Sources/Counter Limited  uplimit=max(derate - 1,0)  tsamp=-1
  Trigger : Outport  VectorParamsAs1DForOutWhenUnconnected=off
  wires:
  Compare To Constant/1 -> Trigger/1
  Counter Limited/1 -> Compare To Constant/1

== system LibDBC_SCU_ch1/mBMS_PP/bit_unpacking1 ==
  Data_in : Inport
  bit_unpacking_s : S-Function  FunctionName=bit_unpacking_s  Parameters=SampleTime,Endianness,Format,Inversion,Startbit,Width_bits,Factor,Offset  SFunctionDeploymentMode=off  EnableBusSupport=off
  Data_out : Outport  VectorParamsAs1DForOutWhenUnconnected=off
  wires:
  Data_in/1 -> bit_unpacking_s/1
  bit_unpacking_s/1 -> Data_out/1

== system LibDBC_SCU_ch1/mBMS_PP/bit_unpacking2 ==
  Data_in : Inport
  bit_unpacking_s : S-Function  FunctionName=bit_unpacking_s  Parameters=SampleTime,Endianness,Format,Inversion,Startbit,Width_bits,Factor,Offset  SFunctionDeploymentMode=off  EnableBusSupport=off
  Data_out : Outport  VectorParamsAs1DForOutWhenUnconnected=off
  wires:
  Data_in/1 -> bit_unpacking_s/1
  bit_unpacking_s/1 -> Data_out/1

== system LibDBC_SCU_ch1/mBMS_PP/bit_unpacking3 ==
  Data_in : Inport
  bit_unpacking_s : S-Function  FunctionName=bit_unpacking_s  Parameters=SampleTime,Endianness,Format,Inversion,Startbit,Width_bits,Factor,Offset  SFunctionDeploymentMode=off  EnableBusSupport=off
  Data_out : Outport  VectorParamsAs1DForOutWhenUnconnected=off
  wires:
  Data_in/1 -> bit_unpacking_s/1
  bit_unpacking_s/1 -> Data_out/1

== system LibDBC_SCU_ch1/mBMS_PP/bit_unpacking4 ==
  Data_in : Inport
  bit_unpacking_s : S-Function  FunctionName=bit_unpacking_s  Parameters=SampleTime,Endianness,Format,Inversion,Startbit,Width_bits,Factor,Offset  SFunctionDeploymentMode=off  EnableBusSupport=off
  Data_out : Outport  VectorParamsAs1DForOutWhenUnconnected=off
  wires:
  Data_in/1 -> bit_unpacking_s/1
  bit_unpacking_s/1 -> Data_out/1

== system LibDBC_SCU_ch1/mBMS_RI_OCV_Approx/IO_CAN_ConfigMsg ==
  IO_CAN_ConfigMsg_s : S-Function  FunctionName=IO_CAN_ConfigMsg_s  Parameters=SampleTime,channel,mode,id_format,id,ac_mask  SFunctionDeploymentMode=off  EnableBusSupport=off
  ErrorCode : Outport  VectorParamsAs1DForOutWhenUnconnected=off
  handle : Outport  Port=2  VectorParamsAs1DForOutWhenUnconnected=off
  wires:
  IO_CAN_ConfigMsg_s/2 -> handle/1
  IO_CAN_ConfigMsg_s/1 -> ErrorCode/1

== system LibDBC_SCU_ch1/mBMS_RI_OCV_Approx/IO_CAN_ReadMsg ==
  handle : Inport
  Enable : EnablePort
  IO_CAN_ReadMsg : IOBlock_Library_TTC580/CAN  Blocks TTC580 IOlib/ReadMsg_CAN/IO_CAN_ReadMsg  SampleTime=-1  ttlib=IO_Blk_Lib_TTC500  ttDescription=IO_CAN_ReadMsg  tt_iolib_version=0.19
      settings: SourceProductName=I/O Blocklibrary for TTC580
  ErrorCode : Outport  VectorParamsAs1DForOutWhenUnconnected=off
  buffer_data : Outport  Port=2  VectorParamsAs1DForOutWhenUnconnected=off
  buffer_length : Outport  Port=3  VectorParamsAs1DForOutWhenUnconnected=off
  buffer_id_format : Outport  Port=4  VectorParamsAs1DForOutWhenUnconnected=off
  buffer_id : Outport  Port=5  VectorParamsAs1DForOutWhenUnconnected=off
  wires:
  IO_CAN_ReadMsg/5 -> buffer_id/1
  IO_CAN_ReadMsg/4 -> buffer_id_format/1
  IO_CAN_ReadMsg/3 -> buffer_length/1
  IO_CAN_ReadMsg/2 -> buffer_data/1
  IO_CAN_ReadMsg/1 -> ErrorCode/1
  handle/1 -> IO_CAN_ReadMsg/1

== system LibDBC_SCU_ch1/mBMS_RI_OCV_Approx/Trigger_Block ==
  Compare To Constant : simulink/Logic and Bit Operations/Compare To Constant  relop===  const=trigger_offset  OutDataTypeStr=boolean  ZeroCross=off
  Counter Limited : simulink/Sources/Counter Limited  uplimit=max(derate - 1,0)  tsamp=-1
  Trigger : Outport  VectorParamsAs1DForOutWhenUnconnected=off
  wires:
  Compare To Constant/1 -> Trigger/1
  Counter Limited/1 -> Compare To Constant/1

== system LibDBC_SCU_ch1/mBMS_RI_OCV_Approx/bit_unpacking1 ==
  Data_in : Inport
  bit_unpacking_s : S-Function  FunctionName=bit_unpacking_s  Parameters=SampleTime,Endianness,Format,Inversion,Startbit,Width_bits,Factor,Offset  SFunctionDeploymentMode=off  EnableBusSupport=off
  Data_out : Outport  VectorParamsAs1DForOutWhenUnconnected=off
  wires:
  Data_in/1 -> bit_unpacking_s/1
  bit_unpacking_s/1 -> Data_out/1

== system LibDBC_SCU_ch1/mBMS_RI_OCV_Approx/bit_unpacking2 ==
  Data_in : Inport
  bit_unpacking_s : S-Function  FunctionName=bit_unpacking_s  Parameters=SampleTime,Endianness,Format,Inversion,Startbit,Width_bits,Factor,Offset  SFunctionDeploymentMode=off  EnableBusSupport=off
  Data_out : Outport  VectorParamsAs1DForOutWhenUnconnected=off
  wires:
  Data_in/1 -> bit_unpacking_s/1
  bit_unpacking_s/1 -> Data_out/1
